simulink model "Park"  (R2014b)
settings: Solver=ode45  StartTime=0.0  StopTime=0.1  RelTol=1e-3
settings Model: Creator=Lei  LastModifiedBy=Lei

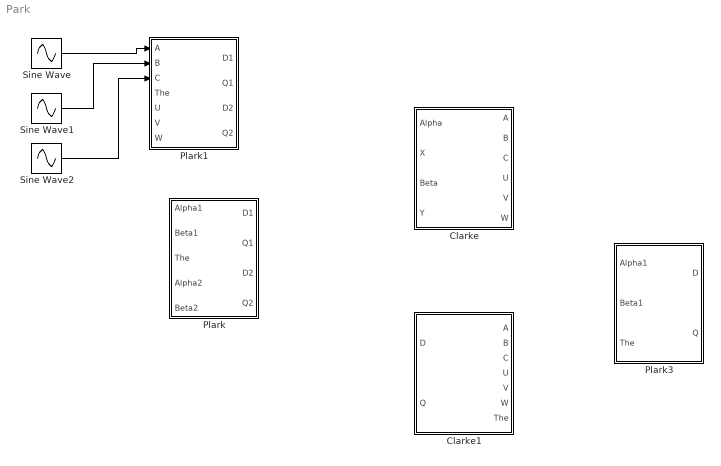
== system Park ==
  Clarke : Subsystem
  Clarke1 : Subsystem
  Plark : Subsystem
  Plark1 : Subsystem
  Plark3 : Subsystem
  Sine Wave : Sin  Amplitude=100  Frequency=2*pi*50  SampleTime=10e-6
  Sine Wave1 : Sin  Amplitude=100  Frequency=2*pi*50  Phase=-2/3*pi  SampleTime=10e-6
  Sine Wave2 : Sin  Amplitude=100  Frequency=2*pi*50  Phase=2/3*pi  SampleTime=10e-6
  wires:
  Sine Wave1/1 -> Plark1/2(B)
  Sine Wave/1 -> Plark1/1(A)
  Sine Wave2/1 -> Plark1/3(C)

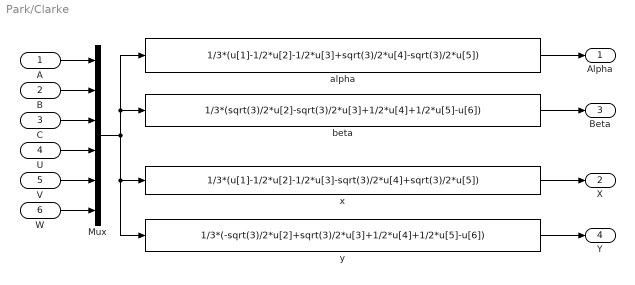
== system Park/Clarke ==
  A : Inport
  B : Inport  Port=2
  C : Inport  Port=3
  U : Inport  Port=4
  V : Inport  Port=5
  W : Inport  Port=6
  Mux : Mux  Inputs=6
  alpha : Fcn  Expr=1/3*(u[1]-1/2*u[2]-1/2*u[3]+sqrt(3)/2*u[4]-sqrt(3)/2*u[5])
  beta : Fcn  Expr=1/3*(sqrt(3)/2*u[2]-sqrt(3)/2*u[3]+1/2*u[4]+1/2*u[5]-u[6])
  x : Fcn  Expr=1/3*(u[1]-1/2*u[2]-1/2*u[3]-sqrt(3)/2*u[4]+sqrt(3)/2*u[5])
  y : Fcn  Expr=1/3*(-sqrt(3)/2*u[2]+sqrt(3)/2*u[3]+1/2*u[4]+1/2*u[5]-u[6])
  Alpha : Outport
  X : Outport  Port=2
  Beta : Outport  Port=3
  Y : Outport  Port=4
  wires:
  Mux/1 -> alpha/1, beta/1, x/1, y/1
  B/1 -> Mux/2
  C/1 -> Mux/3
  A/1 -> Mux/1
  U/1 -> Mux/4
  V/1 -> Mux/5
  W/1 -> Mux/6
  alpha/1 -> Alpha/1
  beta/1 -> Beta/1
  x/1 -> X/1
  y/1 -> Y/1

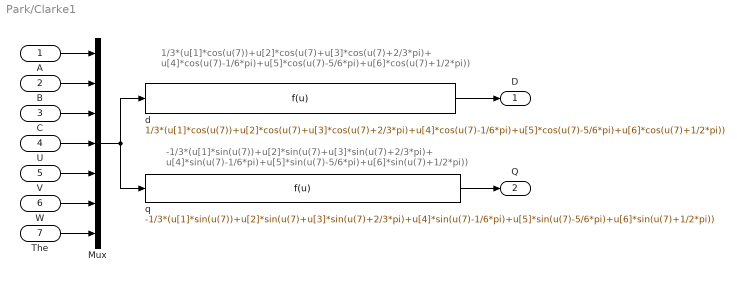
== system Park/Clarke1 ==
  note: -1/3*(u[1]*sin(u(7))+u[2]*sin(u(7)+u[3]*sin(u(7)+2/3*pi)+
      | u[4]*sin(u(7)-1/6*pi)+u[5]*sin(u(7)-5/6*pi)+u[6]*sin(u(7)+1/2*pi))
  note: 1/3*(u[1]*cos(u(7))+u[2]*cos(u(7)+u[3]*cos(u(7)+2/3*pi)+
      | u[4]*cos(u(7)-1/6*pi)+u[5]*cos(u(7)-5/6*pi)+u[6]*cos(u(7)+1/2*pi))
  A : Inport
  B : Inport  Port=2
  C : Inport  Port=3
  U : Inport  Port=4
  V : Inport  Port=5
  W : Inport  Port=6
  The : Inport  Port=7
  Mux : Mux  Inputs=7
  d : Fcn  Expr=1/3*(u[1]*cos(u(7))+u[2]*cos(u(7)+u[3]*cos(u(7)+2/3*pi)+u[4]*cos(u(7)-1/6*pi)+u[5]*cos(u(7)-5/6*pi)+u[6]*cos(u(7)+1/2*pi))
  q : Fcn  Expr=-1/3*(u[1]*sin(u(7))+u[2]*sin(u(7)+u[3]*sin(u(7)+2/3*pi)+u[4]*sin(u(7)-1/6*pi)+u[5]*sin(u(7)-5/6*pi)+u[6]*sin(u(7)+1/2*pi))
  D : Outport
  Q : Outport  Port=2
  wires:
  q/1 -> Q/1
  d/1 -> D/1
  W/1 -> Mux/6
  V/1 -> Mux/5
  U/1 -> Mux/4
  A/1 -> Mux/1
  C/1 -> Mux/3
  B/1 -> Mux/2
  Mux/1 -> q/1, d/1
  The/1 -> Mux/7

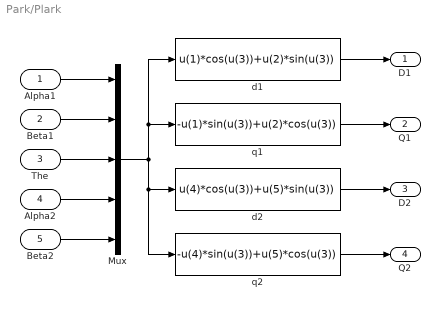
== system Park/Plark ==
  Alpha1 : Inport
  Beta1 : Inport  Port=2
  The : Inport  Port=3
  Alpha2 : Inport  Port=4
  Beta2 : Inport  Port=5
  Mux : Mux  Inputs=5
  d1 : Fcn  Expr=u(1)*cos(u(3))+u(2)*sin(u(3))
  d2 : Fcn  Expr=u(4)*cos(u(3))+u(5)*sin(u(3))
  q1 : Fcn  Expr=-u(1)*sin(u(3))+u(2)*cos(u(3))
  q2 : Fcn  Expr=-u(4)*sin(u(3))+u(5)*cos(u(3))
  D1 : Outport
  Q1 : Outport  Port=2
  D2 : Outport  Port=3
  Q2 : Outport  Port=4
  wires:
  d1/1 -> D1/1
  Beta1/1 -> Mux/2
  The/1 -> Mux/3
  Alpha1/1 -> Mux/1
  q1/1 -> Q1/1
  Alpha2/1 -> Mux/4
  Beta2/1 -> Mux/5
  d2/1 -> D2/1
  q2/1 -> Q2/1
  Mux/1 -> d2/1, q2/1, q1/1, d1/1

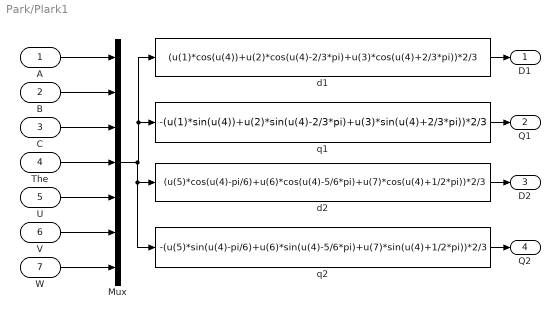
== system Park/Plark1 ==
  A : Inport
  B : Inport  Port=2
  C : Inport  Port=3
  The : Inport  Port=4
  U : Inport  Port=5
  V : Inport  Port=6
  W : Inport  Port=7
  Mux : Mux  Inputs=7
  d1 : Fcn  Expr=(u(1)*cos(u(4))+u(2)*cos(u(4)-2/3*pi)+u(3)*cos(u(4)+2/3*pi))*2/3
  d2 : Fcn  Expr=(u(5)*cos(u(4)-pi/6)+u(6)*cos(u(4)-5/6*pi)+u(7)*cos(u(4)+1/2*pi))*2/3
  q1 : Fcn  Expr=-(u(1)*sin(u(4))+u(2)*sin(u(4)-2/3*pi)+u(3)*sin(u(4)+2/3*pi))*2/3
  q2 : Fcn  Expr=-(u(5)*sin(u(4)-pi/6)+u(6)*sin(u(4)-5/6*pi)+u(7)*sin(u(4)+1/2*pi))*2/3
  D1 : Outport
  Q1 : Outport  Port=2
  D2 : Outport  Port=3
  Q2 : Outport  Port=4
  wires:
  A/1 -> Mux/1
  B/1 -> Mux/2
  d1/1 -> D1/1
  The/1 -> Mux/4
  C/1 -> Mux/3
  q1/1 -> Q1/1
  U/1 -> Mux/5
  V/1 -> Mux/6
  W/1 -> Mux/7
  d2/1 -> D2/1
  q2/1 -> Q2/1
  Mux/1 -> d2/1, q2/1, q1/1, d1/1

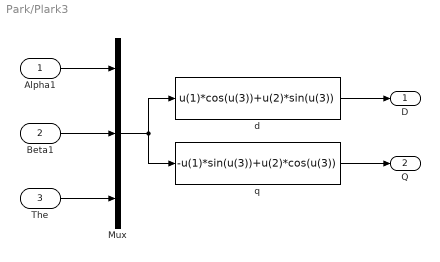
== system Park/Plark3 ==
  Alpha1 : Inport
  Beta1 : Inport  Port=2
  The : Inport  Port=3
  Mux : Mux  Inputs=3
  d : Fcn  Expr=u(1)*cos(u(3))+u(2)*sin(u(3))
  q : Fcn  Expr=-u(1)*sin(u(3))+u(2)*cos(u(3))
  D : Outport
  Q : Outport  Port=2
  wires:
  Mux/1 -> d/1, q/1
  q/1 -> Q/1
  Alpha1/1 -> Mux/1
  The/1 -> Mux/3
  Beta1/1 -> Mux/2
  d/1 -> D/1
